simulink model "exampleTHBCreator"  (R2018b)
settings: Solver=ode45  StartTime=0.0  StopTime=10.0  RelTol=1e-3  EnableMultiTasking=on
libraries: carnot x1
settings Model: Creator=drhf  LastModifiedBy=drhf
settings DataIOCC: LimitDataPoints=on  SaveFormat=Array
settings OptimizationCC: DefaultParameterBehavior=Inlined  LifeSpan=inf
settings DebuggingCC: UnderspecifiedInitializationDetection=Classic  MergeDetectMultiDrivingBlocksExec=none  SolverPrmCheckMsg=warning  SFUnexpectedBacktrackingDiag=warning  SFNoUnconditionalDefaultTransitionDiag=warning  SFExecutionAtInitializationDiag=none
settings HardwareCC: ProdBitPerPointer=32  ProdBitPerSizeT=32  ProdBitPerPtrDiffT=32  ProdLargestAtomicFloat=None  ProdIntDivRoundTo=Undefined  ProdEndianess=Unspecified  ProdWordSize=32  ProdHWDeviceType=32-bit Generic
settings ModelReferenceCC: PropagateSignalLabelsOutOfModel=off
settings SFSimCC: SimUseLocalCustomCode=off
settings RTWCC: RTWUseLocalCustomCode=off
settings CodeAppCC: StateflowObjectComments=on
settings GRTTargetCC: TargetLangStandard=C89/C90 (ANSI)  GeneratePreprocessorConditionals=Disable all
settings ConfigComp: CovMetricSettings=dw  CovHtmlReporting=on  CovSaveCumulativeToWorkspaceVar=on  CovSaveSingleToWorkspaceVar=on  CovExternalEMLEnable=off

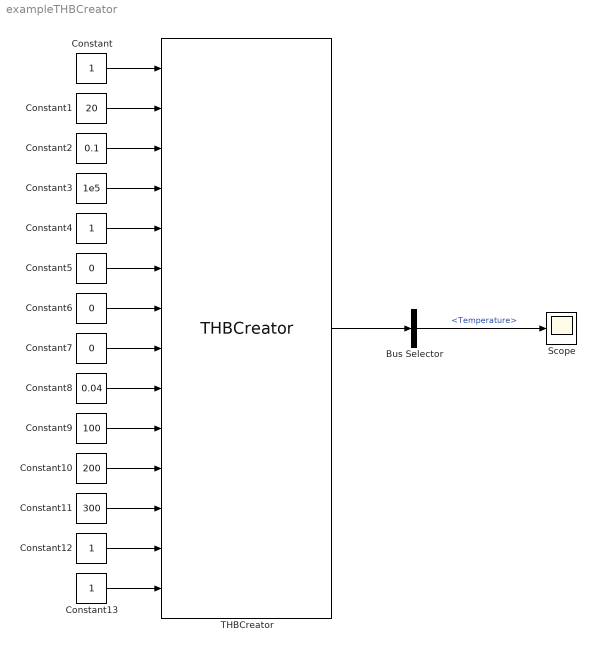
== system exampleTHBCreator ==
  Bus Selector : BusSelector  OutputSignals=Temperature
  Constant{,4,12..13} (4 alike) : Constant
  Constant1 : Constant  Value=20
  Constant10 : Constant  Value=200
  Constant11 : Constant  Value=300
  Constant2 : Constant  Value=0.1
  Constant3 : Constant  Value=1e5
  Constant5 : Constant  Value=0
  Constant6 : Constant  Value=0
  Constant7 : Constant  Value=0
  Constant8 : Constant  Value=0.04
  Constant9 : Constant  Value=100
  Scope : Scope
  THBCreator : carnot/Basic/Hydraulics/THBCreator  Inport_ID=on  Inport_T=on  Inport_mdot=on  Inport_p=on  Inport_type=on  Inport_mix=on  Inport_mix2=on  Inport_mix3=on  Inport_d=on  Inport_c=on  Inport_l=on  Inport_q=on  Inport_LH=on  Inport_H=on  ID=20001  T=20  mdot=0  p=1e5  FluidType=1  FluidMix=0  FluidMix2=0  FluidMix3=0  d=0.02  c=0  l=0  q=0  LH=0  H=0  Annotation_ID=off  Annotation_T=off  Annotation_mdot=off  Annotation_p=off  Annotation_type=off  Annotation_mix=off  Annotation_mix2=off  Annotation_mix3=off  Annotation_d=off  Annotation_c=off  Annotation_l=off  Annotation_q=off  Annotation_LH=off  Annotation_H=off
  wires:
  Constant/1 -> THBCreator/1
  Constant1/1 -> THBCreator/2
  THBCreator/1 -> Bus Selector/1
  Constant2/1 -> THBCreator/3
  Constant3/1 -> THBCreator/4
  Constant4/1 -> THBCreator/5
  Constant5/1 -> THBCreator/6
  Constant6/1 -> THBCreator/7
  Constant7/1 -> THBCreator/8
  Constant8/1 -> THBCreator/9
  Constant9/1 -> THBCreator/10
  Constant10/1 -> THBCreator/11
  Constant11/1 -> THBCreator/12
  Constant12/1 -> THBCreator/13
  Constant13/1 -> THBCreator/14
  Bus Selector/1 -> Scope/1  "<Temperature>"
